simulink model "DF_fixp16_alu_av"  (R2020b)
settings: Solver=ode45  StartTime=0.0  StopTime=0.00001  RelTol=1e-3  EnableMultiTasking=on
PreLoadFcn:
  | setup_DF_fixp16_alu_av;
InitFcn:
  | setup_DF_fixp16_alu_av;
values from neighbouring files (symbols this model uses):
  constwordlength = 32    [setup_DF_fixp16_alu_av.m]    (also in setup_sim_DF_fixp16_alu.m; setup_verify_DF_fixp16_alu.m)
  constwordlengthIn = 16    [setup_DF_fixp16_alu_av.m]    (also in setup_sim_DF_fixp16_alu.m; setup_verify_DF_fixp16_alu.m)
  DSPBASampleTime = FoldingFactor / (ClockFrequency * 1e6)    (= 5e-06)    [setup_DF_fixp16_alu_av.m]    (also in setup_sim_DF_fixp16_alu.m; setup_verify_DF_fixp16_alu.m)
undefined symbols (not defined in the file or in its folder): dpoly, evalAionMaskParam, value
libraries: DSPBAPrim x27, DSPBAModelBus x21, DSPBABase x7, foc_blocks x2
settings Model: Creator=ksmith  LastModifiedBy=mevalver
settings DataIOCC: LimitDataPoints=on  SaveFormat=StructureWithTime  SignalLoggingSaveFormat=ModelDataLogs  ReturnWorkspaceOutputs=off
settings OptimizationCC: ExpressionDepthLimit=2147483647  LifeSpan=inf
settings DebuggingCC: UnderspecifiedInitializationDetection=Classic  MergeDetectMultiDrivingBlocksExec=none  SolverPrmCheckMsg=warning  FcnCallInpInsideContextMsg=warning  AllowSymbolicDim=off  StateNameClashWarn=warning  SFUnexpectedBacktrackingDiag=warning  SFNoUnconditionalDefaultTransitionDiag=warning  SFExecutionAtInitializationDiag=none  ArithmeticOperatorsInVariantConditions=warning
settings HardwareCC: ProdBitPerPointer=32  ProdBitPerSizeT=32  ProdBitPerPtrDiffT=32  ProdLargestAtomicFloat=None  ProdIntDivRoundTo=Undefined  ProdEndianess=Unspecified  ProdWordSize=32  ProdHWDeviceType=32-bit Generic
settings ModelReferenceCC: PropagateSignalLabelsOutOfModel=off
settings SFSimCC: SimUseLocalCustomCode=off  CustomCodeUndefinedFunction=UseInterfaceOnly
settings RTWCC: RTWUseLocalCustomCode=off
settings CodeAppCC: StateflowObjectComments=on
settings GRTTargetCC: TargetLangStandard=C89/C90 (ANSI)  CombineOutputUpdateFcns=off  GRTInterface=on
settings ConfigComp: CovMetricSettings=dw  CovSaveCumulativeToWorkspaceVar=on  CovSaveSingleToWorkspaceVar=on  CovExternalEMLEnable=off

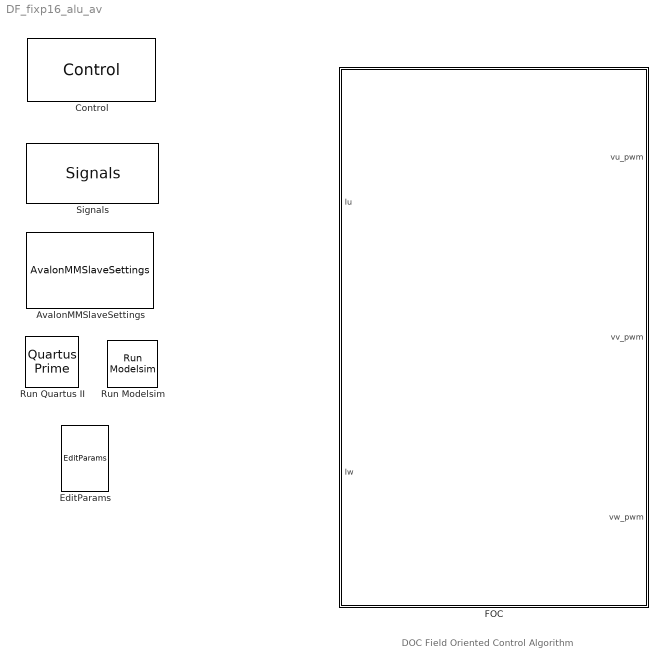
== system DF_fixp16_alu_av ==
  note: DOC Field Oriented Control Algorithm
  AvalonMMSlaveSettings : DSPBABase/AvalonMMSlaveSettings
  Control : DSPBABase/Control  generate=on  language=VHDL  destination=./rtlmax10  destination_gui=./rtlmax10  make_full_path=off  path_is_relative=on  autotestbench=on  signaldepth=2  coveragetestbench=off  logs=off  spacewidth=2  spacenum=1  addrwidth=6  datawidth=32  dataendian=Big Endian  hierarchicalnames=off  ramThresholdBits=-1  distRamThresholdBits=-1  mlabThresholdBits=-1  hardMultiplierThresholdLuts=-1  version=20090407  errorOnChanMismatch=1  errorOnGPIOMismatch=0  importModelsimResults=0  cycleAccurate=off  reinterpretCastMult=off  paramFile=DF_fixp16_alu_av_params.xml
      settings: AttributesFormatString=HDL Generation is %<generate>
  EditParams : DSPBABase/EditParams  version=20090407
  FOC : Subsystem
  Run Modelsim : DSPBABase/Run Modelsim  version=20090407
  Run Quartus II : DSPBABase/Quartus Prime  version=20090407
  Signals : DSPBABase/Signals  clk=clk  freq=ClockFrequency  margin=0  rst=areset  rstactive=High  bus=bus  enbusclock=off  busfreq=100  bussync=on  version=20090407

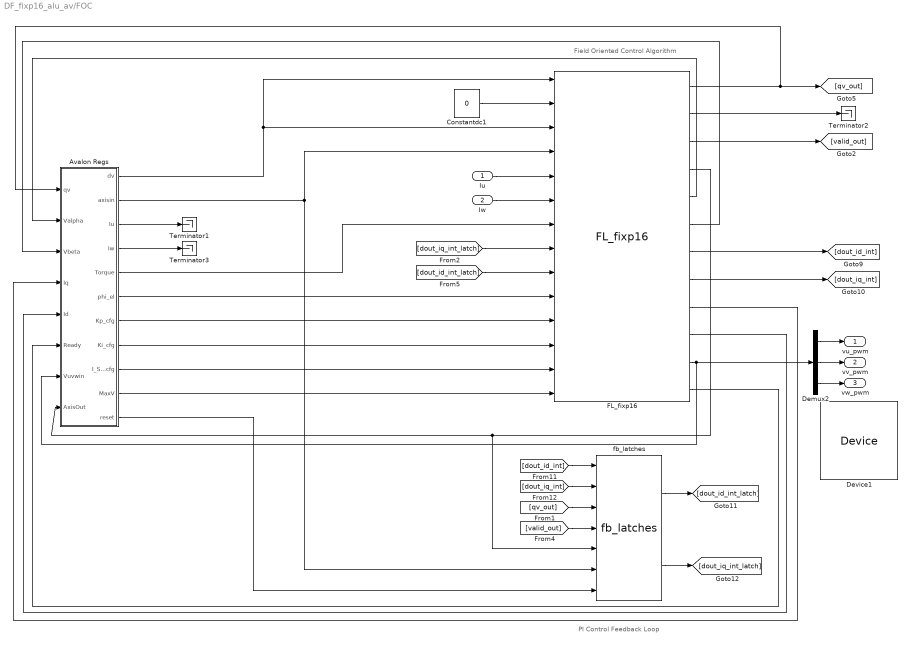
== system DF_fixp16_alu_av/FOC ==
  note: Field Oriented Control Algorithm
  note: PI Control Feedback Loop
  Iu : Inport  OutDataTypeStr=fixdt(1,16,10)
  Iw : Inport  Port=2  OutDataTypeStr=fixdt(1,16,10)
  Avalon Regs : Subsystem
  Constantdc1 : Constant  Value=0  OutDataTypeStr=uint8  SampleTime=DSPBASampleTime
  Demux2 : Demux  Outputs=3
  Device1 : DSPBABase/Device  family=MAX 10  deviceMember=Stratix V GX  stratix4device=Stratix IV E  hardcopy4device=HardCopy IV E  stratix5device=Stratix V GX  device=AUTO  speed=6  stratixSpeed=-5  stratix2Speed=-3  stratix3Speed=-2  stratix4gxSpeed=-2  stratix4gtSpeed=-1  cyclone2Speed=-6  cyclone3Speed=-7  arria2Speed=-4  cyclone4eSpeed=-8  stratix5Speed=-3  arria5Speed=-4  arriaSpeed=-6  cyclone3lsSpeed=-7  cyclone5Speed=-6  arria2gzSpeed=-3  nightFurySpeed=-2  ecp2Speed=-7  hardcopycompat=off  version=20140217  max10flashmode=off  max10nomeminit=off
  FL_fixp16 : foc_blocks/FL_fixp16  SystemSampleTime=-1  VariantActivationTime=update diagram  Latency=0  AutoFrameSizeCalculation=off
      link override ChannelOut1: latency=33
      settings: SourceProductName=FOC Blocks
  Terminator1 : Terminator
  Terminator2 : Terminator
  Terminator3 : Terminator
  fb_latches : foc_blocks/fb_latches  SystemSampleTime=-1  VariantActivationTime=update diagram  Latency=0  AutoFrameSizeCalculation=off
      link override GPOut1: latency=1
      link override GPOut2: latency=1
      settings: SourceProductName=FOC Blocks
  vu_pwm : Outport
  vv_pwm : Outport  Port=2
  vw_pwm : Outport  Port=3
  wires:
  Avalon Regs/6(phi_el) -> FL_fixp16/10
  FL_fixp16/9 -> Avalon Regs/4(Iq)
  Avalon Regs/11(reset) -> fb_latches/7
  Avalon Regs/7(Kp_cfg) -> FL_fixp16/11
  FL_fixp16/4 -> fb_latches/5, Avalon Regs/8(AxisOut)
  FL_fixp16/2 -> Terminator2/1
  Avalon Regs/9(I_Sat_Limit_cfg) -> FL_fixp16/13
  fb_latches/2 -> [dout_iq_int_latch]
  FL_fixp16/3 -> [valid_out]
  FL_fixp16/1 -> [qv_out], Avalon Regs/1(qv)
  fb_latches/1 -> [dout_id_int_latch]
  FL_fixp16/10 -> Avalon Regs/5(Id)
  FL_fixp16/6 -> Avalon Regs/3(Vbeta)
  Avalon Regs/2(axisin) -> FL_fixp16/4, fb_latches/6
  Avalon Regs/10(MaxV) -> FL_fixp16/14
  FL_fixp16/12 -> Avalon Regs/6(Ready)
  [qv_out] -> fb_latches/3
  FL_fixp16/8 -> [dout_iq_int]
  Avalon Regs/1(dv) -> FL_fixp16/1, FL_fixp16/3
  Avalon Regs/5(Torque) -> FL_fixp16/7
  [dout_id_int] -> fb_latches/1
  [dout_iq_int_latch] -> FL_fixp16/8
  FL_fixp16/11 -> Demux2/1, Avalon Regs/7(Vuvwin)
  [dout_id_int_latch] -> FL_fixp16/9
  Avalon Regs/8(Ki_cfg) -> FL_fixp16/12
  [valid_out] -> fb_latches/4
  [dout_iq_int] -> fb_latches/2
  FL_fixp16/7 -> [dout_id_int]
  FL_fixp16/5 -> Avalon Regs/2(Valpha)
  Constantdc1/1 -> FL_fixp16/2
  Iw/1 -> FL_fixp16/6
  Iu/1 -> FL_fixp16/5
  Avalon Regs/3(Iu) -> Terminator1/1
  Avalon Regs/4(Iw) -> Terminator3/1
  Demux2/1 -> vu_pwm/1
  Demux2/3 -> vw_pwm/1
  Demux2/2 -> vv_pwm/1

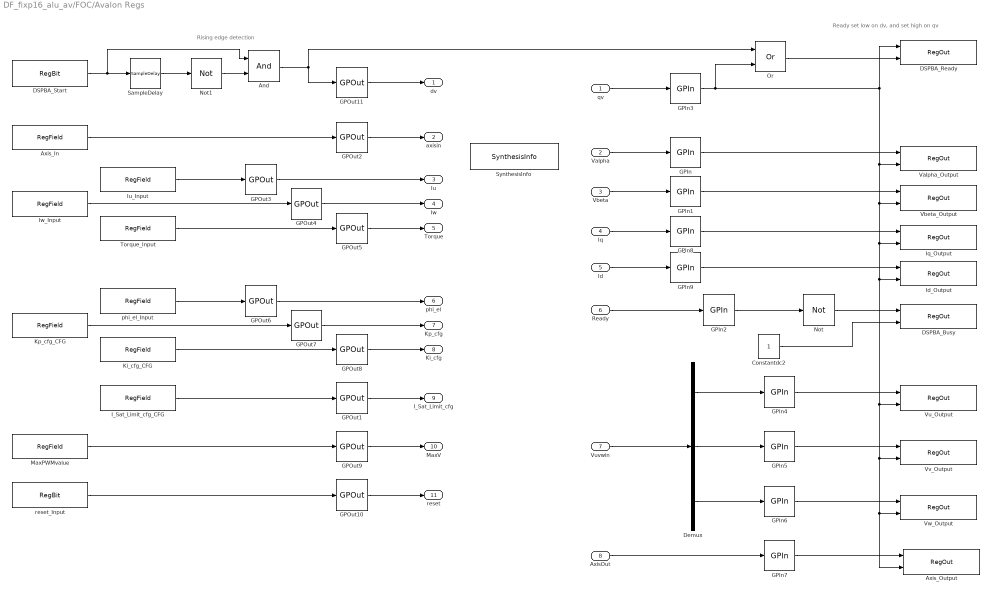
== system DF_fixp16_alu_av/FOC/Avalon Regs ==
  note: Rising edge detection
  note: Ready set low on dv, and set high on qv
  qv : Inport
  Valpha : Inport  Port=2
  Vbeta : Inport  Port=3
  Iq : Inport  Port=4
  Id : Inport  Port=5
  Ready : Inport  Port=6
  Vuvwin : Inport  Port=7
  AxisOut : Inport  Port=8
  And : DSPBAPrim/And  primtype=and  nInputs=2  nOutputs=1  omode=Inherit via internal rule  otype=sfix(16)  scale=2^-15  rndmethod=Unbiased  factor=1  satmethod=Symmetric  shift_vec=[0 1 2 -1]  value=0  inPortNames=[' '; ' '; ' '; ' '; ' '; ' '; ' '; ' '; ' '; ' '; ' '; ' '; ' '; ' '; ' '; ' '; ]  outPortNames=[' ']  dspbaimage=dspba_prim.svg  text=fprintf('&');  style=Optimised  visibilities=8+2  version=20211007
  Axis_In : DSPBAModelBus/RegField  reg_name=Axis  reg_rwmode=Read/Write  reg_msb=7  reg_lsb=0  reg_mode=Specify via dialog  reg_type=uint(8)  reg_scale=0  reg_init=0  reg_desc=Dummy - not used. Set to 0.  reg_modal=off  reg_desc0=0  reg_desc1=0  reg_desc2=0  reg_desc3=0  reg_desc4=0  reg_desc5=0  reg_desc6=0  reg_desc7=0  reg_addr=2  SampleTime=DSPBASampleTime  version=20090407
  Axis_Output : DSPBAModelBus/RegOut  reg_name=AxisReg  reg_rwmode=Read  reg_msb=7  reg_lsb=0  reg_desc=Axis value  reg_addr=60  SampleTime=-1  version=20090407
  Constantdc2 : Constant  OutDataTypeStr=boolean  SampleTime=DSPBASampleTime
  DSPBA_Busy : DSPBAModelBus/RegOut  reg_name=Busy  reg_rwmode=Read  reg_msb=0  reg_lsb=0  reg_desc=Busy bit - When '1' not ready to accept new data  reg_addr=0  SampleTime=-1  version=20090407
  DSPBA_Ready : DSPBAModelBus/RegOut  reg_name=Ready  reg_rwmode=Read  reg_msb=0  reg_lsb=0  reg_desc=Ready bit - Output data is ready when 'Control' reg value matches 'Ready'  reg_addr=3  SampleTime=-1  version=20090407
  DSPBA_Start : DSPBAModelBus/RegBit  reg_name=Start  reg_rwmode=Read/Write  reg_lsb=0  reg_init=0  reg_desc=Start bit - toggle bit value once to start  reg_addr=1  reg_desc0=0  reg_desc1=0  SampleTime=DSPBASampleTime  version=20090407
  Demux : Demux  Outputs=3
  GPIn{,1..9} (10 alike) : DSPBAPrim/GPIn  primtype=gpin  nInputs=evalAionMaskParam(gcb,'value',1)  nOutputs=evalAionMaskParam(gcb,'value',1)  omode=Inherit via internal rule  otype=sfix(16)  scale=2^-15  rndmethod=Unbiased  factor=1  satmethod=Symmetric  shift_vec=[0 1 2 -1]  value=1  inPortNames=[' ' ' ' ' ' ' ' ' ' ' ' ' ' ' ' ' ' ' ' ' ' ' ' ' ' ' ' ' ' ' ' ' ' ' ' ' ' ' ' ' ' ' ' ' ' ' ' ' ' ' ' ' ' ' ' ' ' ' ' ' ' ' ' ' ' ' ' ' ']'  outPortNames=[' ' ' ' ' ' ' ' ' ' ' ' ' ' ' ' ' ' ' ' ' ' ' ' ' ' ' ' ' ' ' ' ' ' ' ' ' ' ' ' ' ' ' ' ' ' ' ' ' ' ' ' ' ' ' ' ' ' ' ' ' ' ' ' ' ' ' ' ' ']'  dspbaimage=dspba_prim_channel_tall.svg  text=fprintf('GPIn');  style=Optimised  visibilities=1024  scheduleOrigin=off  version=20211214
  GPOut{1..10} (10 alike) : DSPBAPrim/GPOut  primtype=gpout  nInputs=evalAionMaskParam(gcb,'value',1)  nOutputs=evalAionMaskParam(gcb,'value',1)  omode=Inherit via internal rule  otype=sfix(16)  scale=2^-15  rndmethod=Unbiased  factor=1  satmethod=Symmetric  shift_vec=[0 1 2 -1]  value=1  inPortNames=[' ' ' ' ' ' ' ' ' ' ' ' ' ' ' ' ' ' ' ' ' ' ' ' ' ' ' ' ' ' ' ' ' ' ' ' ' ' ' ' ' ' ' ' ' ' ' ' ' ' ' ' ' ' ' ' ' ' ' ' ' ' ' ' ' ' ' ' ' ']'  outPortNames=[' ' ' ' ' ' ' ' ' ' ' ' ' ' ' ' ' ' ' ' ' ' ' ' ' ' ' ' ' ' ' ' ' ' ' ' ' ' ' ' ' ' ' ' ' ' ' ' ' ' ' ' ' ' ' ' ' ' ' ' ' ' ' ' ' ' ' ' ' ']'  dspbaimage=dspba_prim_channel_tall.svg  text=fprintf('GPOut');  style=Optimised  visibilities=1024  latency=0  version=20211214
  GPOut11 : DSPBAPrim/GPOut  primtype=gpout  nInputs=evalAionMaskParam(gcb,'value',1)  nOutputs=evalAionMaskParam(gcb,'value',1)  omode=Inherit via internal rule  otype=sfix(16)  scale=2^-15  rndmethod=Unbiased  factor=1  satmethod=Symmetric  shift_vec=[0 1 2 -1]  value=1  inPortNames=[' ' ' ' ' ' ' ' ' ' ' ' ' ' ' ' ' ' ' ' ' ' ' ' ' ' ' ' ' ' ' ' ' ' ' ' ' ' ' ' ' ' ' ' ' ' ' ' ' ' ' ' ' ' ' ' ' ' ' ' ' ' ' ' ' ' ' ' ' ']'  outPortNames=[' ' ' ' ' ' ' ' ' ' ' ' ' ' ' ' ' ' ' ' ' ' ' ' ' ' ' ' ' ' ' ' ' ' ' ' ' ' ' ' ' ' ' ' ' ' ' ' ' ' ' ' ' ' ' ' ' ' ' ' ' ' ' ' ' ' ' ' ' ']'  dspbaimage=dspba_prim_channel_tall.svg  text=fprintf('GPOut');  style=Optimised  visibilities=1024  latency=1  version=20211214
  I_Sat_Limit_cfg_CFG : DSPBAModelBus/RegField  reg_name=I_Sat_Limit_cfg  reg_rwmode=Read/Write  reg_msb=constwordlengthIn-1  reg_lsb=0  reg_mode=Specify via dialog  reg_type=constOTypeIn  reg_scale=constScaleIn  reg_init=0  reg_desc=I_Sat_Limit_cfg input value  reg_modal=off  reg_desc0=0  reg_desc1=0  reg_desc2=0  reg_desc3=0  reg_desc4=0  reg_desc5=0  reg_desc6=0  reg_desc7=0  reg_addr=19  SampleTime=DSPBASampleTime  version=20090407
  Id_Output : DSPBAModelBus/RegOut  reg_name=xId  reg_rwmode=Read  reg_msb=constwordlengthIn-1  reg_lsb=0  reg_desc=Id output value  reg_addr=55  SampleTime=-1  version=20090407
  Iq_Output : DSPBAModelBus/RegOut  reg_name=xIq  reg_rwmode=Read  reg_msb=constwordlengthIn-1  reg_lsb=0  reg_desc=Iq output value  reg_addr=54  SampleTime=-1  version=20090407
  Iu_Input : DSPBAModelBus/RegField  reg_name=Iu  reg_rwmode=Read/Write  reg_msb=constwordlengthIn-1  reg_lsb=0  reg_mode=Specify via dialog  reg_type=constOTypeIn  reg_scale=constScaleIn  reg_init=0  reg_desc=Iu input value  reg_modal=off  reg_desc0=0  reg_desc1=0  reg_desc2=0  reg_desc3=0  reg_desc4=0  reg_desc5=0  reg_desc6=0  reg_desc7=0  reg_addr=32  SampleTime=DSPBASampleTime  version=20090407
  Iw_Input : DSPBAModelBus/RegField  reg_name=Iw  reg_rwmode=Read/Write  reg_msb=constwordlengthIn-1  reg_lsb=0  reg_mode=Specify via dialog  reg_type=constOTypeIn  reg_scale=constScaleIn  reg_init=0  reg_desc=Iw input value  reg_modal=off  reg_desc0=0  reg_desc1=0  reg_desc2=0  reg_desc3=0  reg_desc4=0  reg_desc5=0  reg_desc6=0  reg_desc7=0  reg_addr=33  SampleTime=DSPBASampleTime  version=20090407
  Ki_cfg_CFG : DSPBAModelBus/RegField  reg_name=Ki_cfg  reg_rwmode=Read/Write  reg_msb=constwordlengthIn-1  reg_lsb=0  reg_mode=Specify via dialog  reg_type=constOTypeIn  reg_scale=constScaleIn  reg_init=0  reg_desc=Ki_cfg input value  reg_modal=off  reg_desc0=0  reg_desc1=0  reg_desc2=0  reg_desc3=0  reg_desc4=0  reg_desc5=0  reg_desc6=0  reg_desc7=0  reg_addr=17  SampleTime=DSPBASampleTime  version=20090407
  Kp_cfg_CFG : DSPBAModelBus/RegField  reg_name=Kp_cfg  reg_rwmode=Read/Write  reg_msb=constwordlengthIn-1  reg_lsb=0  reg_mode=Specify via dialog  reg_type=constOTypeIn  reg_scale=constScaleIn  reg_init=0  reg_desc=Kp_cfg input value  reg_modal=off  reg_desc0=0  reg_desc1=0  reg_desc2=0  reg_desc3=0  reg_desc4=0  reg_desc5=0  reg_desc6=0  reg_desc7=0  reg_addr=16  SampleTime=DSPBASampleTime  version=20090407
  MaxPWMvalue : DSPBAModelBus/RegField  reg_name=MaximumVreg  reg_rwmode=Read/Write  reg_msb=15  reg_lsb=0  reg_mode=Specify via dialog  reg_type=uint(16)  reg_scale=2^-0  reg_init=18750  reg_desc=Maximum Voltage  reg_modal=off  reg_desc0=0  reg_desc1=0  reg_desc2=0  reg_desc3=0  reg_desc4=0  reg_desc5=0  reg_desc6=0  reg_desc7=0  reg_addr=62  SampleTime=DSPBASampleTime  version=20090407
  Not : DSPBAPrim/Not  primtype=not  nInputs=1  nOutputs=1  omode=Inherit via internal rule  otype=sfix(16)  scale=2^-15  rndmethod=Unbiased  factor=1  satmethod=Symmetric  shift_vec=[0 1 2 -1]  value=0  inPortNames=[' '; ' ';]  outPortNames=[' ']  dspbaimage=dspba_prim.svg  text=fprintf('~');  style=Optimised  visibilities=8  version=20211007
  Not1 : DSPBAPrim/Not  primtype=not  nInputs=1  nOutputs=1  omode=Inherit via internal rule  otype=sfix(16)  scale=2^-15  rndmethod=Unbiased  factor=1  satmethod=Symmetric  shift_vec=[0 1 2 -1]  value=0  inPortNames=[' '; ' ';]  outPortNames=[' ']  dspbaimage=dspba_prim.svg  text=fprintf('~');  style=Optimised  visibilities=8  version=20211007
  Or : DSPBAPrim/Or  primtype=or  nInputs=2  nOutputs=1  omode=Inherit via internal rule  otype=sfix(16)  scale=2^-15  rndmethod=Unbiased  factor=1  satmethod=Symmetric  shift_vec=[0 1 2 -1]  value=0  inPortNames=[' '; ' '; ' '; ' '; ' '; ' '; ' '; ' '; ' '; ' '; ' '; ' '; ' '; ' '; ' '; ' '; ]  outPortNames=[' ']  dspbaimage=dspba_prim.svg  text=fprintf('|');  style=Optimised  visibilities=8+2  version=20211007
  SampleDelay : DSPBAPrim/SampleDelay  primtype=sampdelay  nInputs=1  nOutputs=1  omode=Inherit via internal rule  otype=sfix(16)  scale=2^-15  rndmethod=Unbiased  factor=1  satmethod=Symmetric  shift_vec=[0 1 2 -1]  floatPrecision=float32_m23  value=1  inPortNames=[' '; ' ';]  outPortNames=[' ']  dspbaimage=dspba_prim.svg  text=dpoly(1, eye(1,value+1), 'z')  style=Optimised  visibilities=8 + 1024 + 2^17 + 2^18  flexible=off  slackgroup=0  augmented=0  version=20211007  advOptions=[]
  SynthesisInfo : DSPBAPrim/SynthesisInfo  primtype=synthinfo  nInputs=0  nOutputs=0  omode=Inherit via internal rule  otype=sfix(16)  scale=2^-15  rndmethod=Truncate  factor=1  satmethod=Symmetric  shift_vec=[0 1 2 -1]  value=99  inPortNames=[' '; ' ';]  outPortNames=[' ']  dspbaimage=dspba_prim_ctrl.jpg  text=fprintf('Style=%s', style);  style=Scheduled  visibilities=32768  constraintPair=None  constraintRelation=>  constraintLimit=2  modelRefSign=+  modelRef=''  showSchedule=off  simulationMode=Use Global Value  resetMinimization=Conditional - On for ChannelIn/Out only  version=20220106
  Torque_Input : DSPBAModelBus/RegField  reg_name=Torque  reg_rwmode=Read/Write  reg_msb=constwordlengthIn-1  reg_lsb=0  reg_mode=Specify via dialog  reg_type=constOTypeIn  reg_scale=constScaleIn  reg_init=0  reg_desc=Torque input value  reg_modal=off  reg_desc0=0  reg_desc1=0  reg_desc2=0  reg_desc3=0  reg_desc4=0  reg_desc5=0  reg_desc6=0  reg_desc7=0  reg_addr=34  SampleTime=DSPBASampleTime  version=20090407
  Valpha_Output : DSPBAModelBus/RegOut  reg_name=Valpha  reg_rwmode=Read  reg_msb=constwordlength-1  reg_lsb=0  reg_desc=Valpha output value  reg_addr=48  SampleTime=-1  version=20090407
  Vbeta_Output : DSPBAModelBus/RegOut  reg_name=Vbeta  reg_rwmode=Read  reg_msb=constwordlength-1  reg_lsb=0  reg_desc=Vbeta output value  reg_addr=49  SampleTime=-1  version=20090407
  Vu_Output : DSPBAModelBus/RegOut  reg_name=VuReg  reg_rwmode=Read  reg_msb=15  reg_lsb=0  reg_desc=Vu output value  reg_addr=56  SampleTime=-1  version=20090407
  Vv_Output : DSPBAModelBus/RegOut  reg_name=VvReg  reg_rwmode=Read  reg_msb=15  reg_lsb=0  reg_desc=Vv output value  reg_addr=57  SampleTime=-1  version=20090407
  Vw_Output : DSPBAModelBus/RegOut  reg_name=VwReg  reg_rwmode=Read  reg_msb=15  reg_lsb=0  reg_desc=Vw output value  reg_addr=58  SampleTime=-1  version=20090407
  phi_el_Input : DSPBAModelBus/RegField  reg_name=phi_el  reg_rwmode=Read/Write  reg_msb=constwordlengthIn-1  reg_lsb=0  reg_mode=Specify via dialog  reg_type=ufix(16)  reg_scale=2^-16  reg_init=0  reg_desc=phi_el input value  reg_modal=off  reg_desc0=0  reg_desc1=0  reg_desc2=0  reg_desc3=0  reg_desc4=0  reg_desc5=0  reg_desc6=0  reg_desc7=0  reg_addr=35  SampleTime=DSPBASampleTime  version=20090407
  reset_Input : DSPBAModelBus/RegBit  reg_name=reset  reg_rwmode=Read/Write  reg_lsb=0  reg_init=0  reg_desc=reset - set to '1' to reset  reg_addr=36  reg_desc0=0  reg_desc1=0  SampleTime=DSPBASampleTime  version=20090407
  dv : Outport
  axisin : Outport  Port=2
  Iu : Outport  Port=3
  Iw : Outport  Port=4
  Torque : Outport  Port=5
  phi_el : Outport  Port=6
  Kp_cfg : Outport  Port=7
  Ki_cfg : Outport  Port=8
  I_Sat_Limit_cfg : Outport  Port=9
  MaxV : Outport  Port=10
  reset : Outport  Port=11
  wires:
  Iw_Input/1 -> GPOut4/1
  Not1/1 -> And/2
  SampleDelay/1 -> Not1/1
  Torque_Input/1 -> GPOut5/1
  Kp_cfg_CFG/1 -> GPOut7/1
  Iu_Input/1 -> GPOut3/1
  Axis_In/1 -> GPOut2/1
  phi_el_Input/1 -> GPOut6/1
  Ki_cfg_CFG/1 -> GPOut8/1
  DSPBA_Start/1 -> And/1, SampleDelay/1
  Or/1 -> DSPBA_Ready/2
  GPOut11/1 -> dv/1
  And/1 -> GPOut11/1, Or/1
  GPOut2/1 -> axisin/1
  GPOut4/1 -> Iw/1
  Constantdc2/1 -> DSPBA_Busy/2
  Valpha/1 -> GPIn/1
  GPOut3/1 -> Iu/1
  GPOut6/1 -> phi_el/1
  Vbeta/1 -> GPIn1/1
  Not/1 -> DSPBA_Busy/1
  GPOut5/1 -> Torque/1
  qv/1 -> GPIn3/1
  GPOut7/1 -> Kp_cfg/1
  Ready/1 -> GPIn2/1
  GPOut8/1 -> Ki_cfg/1
  I_Sat_Limit_cfg_CFG/1 -> GPOut1/1
  GPIn/1 -> Valpha_Output/1
  GPIn1/1 -> Vbeta_Output/1
  GPIn2/1 -> Not/1
  GPOut1/1 -> I_Sat_Limit_cfg/1
  Iq/1 -> GPIn8/1
  Id/1 -> GPIn9/1
  GPIn3/1 -> DSPBA_Ready/1, Valpha_Output/2, Axis_Output/2, Vw_Output/2, Vv_Output/2, Vu_Output/2, Id_Output/2, Iq_Output/2, Vbeta_Output/2, Or/2
  GPIn8/1 -> Iq_Output/1
  GPIn9/1 -> Id_Output/1
  MaxPWMvalue/1 -> GPOut9/1
  GPOut9/1 -> MaxV/1
  GPIn4/1 -> Vu_Output/1
  Vuvwin/1 -> Demux/1
  Demux/1 -> GPIn4/1
  Demux/2 -> GPIn5/1
  Demux/3 -> GPIn6/1
  GPIn5/1 -> Vv_Output/1
  GPIn6/1 -> Vw_Output/1
  AxisOut/1 -> GPIn7/1
  GPIn7/1 -> Axis_Output/1
  GPOut10/1 -> reset/1
  reset_Input/1 -> GPOut10/1
